simulink model "Citation"  (Simulink 9.1)
settings: Solver=ode5  StartTime=0.0  StopTime=100  FixedStep=0.01  RelTol=1e-3  EnableMultiTasking=on
values from neighbouring files (symbols this model uses):
  T0 = 288.15    [rho_test.m]
  Vw915 = 0    [initcit.m]
  winddir = 45*(pi/180)    (= 0.785398163397)    [initcit.m]
  x0 = []    [cessnac550_3d_sfnc.m]    (also in sfunxyauto.m)
undefined symbols (not defined in the file or in its folder): chord, cv1, cv2, cv3, cv4, deltagmax1, deltagmax2, deltagmax3, deltagmax4, Deng, ealphag, ealphas, g0, hDME, hGS, kt1, kt2, kt3, lh, massinit, matbuaf, matdaf, matdam, matdbbf, matdeaf, matdgaf, matdqaf, matduaf, matdwaw, matedhr, mateif, matelhr, matemhr, matemv1, matemv2, matemve, matetam, mateuaf, matfaaf, matfaxl, matff, matibaf, matibmh, matipaf, matipmh, matiraf, matiuaf, matiwaf, matlaf, matlam, matleaf, matleam, matlgaf, matlqaf, matluaf, matmaaf, matmaam, matmaf, matmam, matmbbf ... (+74)
undefined symbols (not defined in the file): matibb
libraries: vrlib x1
(part 1 of 4)
settings Model: Creator=laurensvaneykeren  LastModifiedBy=jelle  ExtModeTrigMode=oneshot  ExtModeArmWhenConnect=off
settings DataIOCC: SignalLoggingSaveFormat=ModelDataLogs  SignalLoggingName=sigsOut
settings OptimizationCC: BooleanDataType=off  ExpressionDepthLimit=2147483647
settings DebuggingCC: SaveWithParameterizedLinksMsg=none  SignalResolutionControl=TryResolveAllWithWarning  MultiTaskDSMMsg=warning  MultiTaskCondExecSysMsg=none  FcnCallInpInsideContextMsg=warning  StateNameClashWarn=warning
settings HardwareCC: TargetUnknown=on
settings RTWCC: SystemTargetFile=grt_malloc.tlc  GenCodeOnly=on  TemplateMakefile=grt_malloc_default_tmf
settings GRTTargetCC: UseMalloc=on

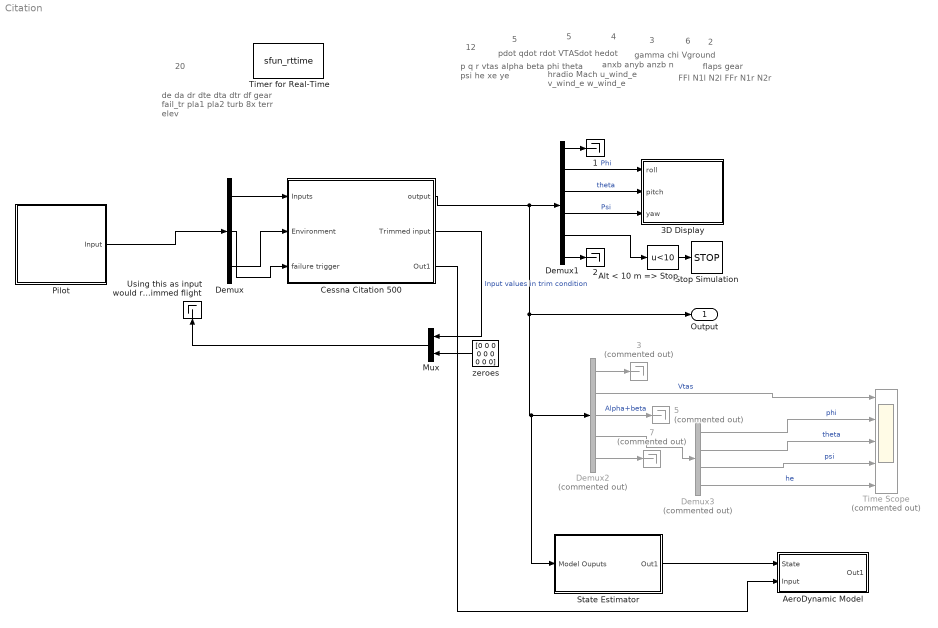
== system Citation ==
  note: de
      | da
      | dr
      | dte
      | dta
      | dtr
      | df
      | gear
      | fail_tr
      | pla1
      | pla2
      | turb 8x
      | terr elev
  note: p
      | q
      | r
      | vtas
      | alpha
      | beta
      | phi
      | theta
      | psi
      | he
      | xe
      | ye
  note: pdot
      | qdot
      | rdot
      | VTASdot
      | hedot
  note: hradio
      | Mach
      | u_wind_e
      | v_wind_e
      | w_wind_e
  note: anxb
      | anyb
      | anzb
      | n
  note: gamma
      | chi
      | Vground
  note: flaps
      | gear
  note: FFl
      | N1l
      | N2l
      | FFr
      | N1r
      | N2r
  note: 12
  note: 5
  note: 5
  note: 4
  note: 3
  note: 6
  note: 2
  note: 20
  1 : Terminator
  2 : Terminator
  3 : Terminator  Commented=on
  3D Display : Subsystem
  5 : Terminator  Commented=on
  7 : Terminator  Commented=on
  "AeroDynamic Model " : Subsystem
  Alt < 10 m => Stop : Fcn  Expr=u<10
  Cessna Citation 500 : Subsystem  mask(Citation Aircraft Model){trimdatafile=example.tri}
      mask prompts: trimdatafile "Trim Condition"
      mask init:
      | initcit;
      mask Display:
      | image(imread('Citation.jpg'))
      | port_label('input', 1, 'Inputs')
      | port_label('input', 2, 'Environment')
      | port_label('output', 1, 'Outputs')
      | port_label('output', 2, 'Trim inputs')
  Demux : Demux  Outputs=[10 1 9]
  Demux1 : Demux  Outputs=[6 1 1 1 1 27]
  Demux2 : Demux  Commented=on  Outputs=[3 1 2 4 27]
  Demux3 : Demux  Commented=on
  Mux : Mux  Inputs=2
  Pilot : Subsystem
  "State Estimator " : Subsystem
  Stop Simulation : Stop
  Time Scope : Scope  Commented=on  NumInputPorts=5
  Timer for Real-Time : S-Function  FunctionName=sfun_rttime  Parameters=1  SFunctionDeploymentMode=off  EnableBusSupport=off
  Using this as input would result in  trimmed flight : Terminator
  zeroes : Constant  Value=[0 0 0 0 0 0 0 0 0]
  Output : Outport
  wires:
  Demux/1 -> Cessna Citation 500/1(Inputs)
  Pilot/1(Input) -> Demux/1
  Cessna Citation 500/1(output) -> Demux1/1, "State Estimator "/1(Model Ouputs), Demux2/1, Output/1
  Demux/3 -> Cessna Citation 500/2(Environment)
  Cessna Citation 500/2(Trimmed input) -> Mux/1  "Input values in trim condition"
  zeroes/1 -> Mux/2
  Mux/1 -> Using this as input would result in  trimmed flight/1
  Demux1/1 -> 1/1
  Demux1/5 -> Alt < 10 m => Stop/1
  Demux1/2 -> 3D Display/1(roll)  "Phi"
  Demux1/3 -> 3D Display/2(pitch)  "theta"
  Demux1/4 -> 3D Display/3(yaw)  "Psi"
  Alt < 10 m => Stop/1 -> Stop Simulation/1
  Demux1/6 -> 2/1
  Demux/2 -> Cessna Citation 500/3("failure trigger ")
  Demux2/1 -> 3/1
  Demux2/2 -> Time Scope/1  "Vtas"
  Demux2/3 -> 5/1  "Alpha+beta"
  Demux2/4 -> Demux3/1
  Demux2/5 -> 7/1
  Demux3/1 -> Time Scope/2  "phi"
  Demux3/2 -> Time Scope/3  "theta"
  Demux3/3 -> Time Scope/4  "psi"
  Demux3/4 -> Time Scope/5  "he"
  "State Estimator "/1(Out1) -> "AeroDynamic Model "/1(State)
  Cessna Citation 500/3(Out1) -> "AeroDynamic Model "/2(Input)

== system Citation/3D Display ==
  roll : Inport
  pitch : Inport  Port=2
  yaw : Inport  Port=3
  Mux1 : Mux
  Position : Subsystem
  S-Function : S-Function  FunctionName=cessnac550_3d_sfnc  SFunctionDeploymentMode=off  EnableBusSupport=off
  Stop Simulation : Stop
  wires:
  roll/1 -> Mux1/1
  Position/1(Out1) -> Mux1/4
  pitch/1 -> Mux1/2
  yaw/1 -> Mux1/3
  Mux1/1 -> S-Function/1
  S-Function/1 -> Stop Simulation/1

== system Citation/AeroDynamic Model  ==
  note: anxb
      | anyb
      | anzb
      | n
  note: hradio
      | Mach
      | u_wind_e
      | v_wind_e
      | w_wind_e
  note: p
      | q
      | r
      | vtas
      | alpha
      | beta
      | phi
      | theta
      | psi
      | he
      | xe
      | ye
  note: gamma
      | chi
      | Vground
  note: pdot
      | qdot
      | rdot
      | VTASdot
      | hedot
  note: FFl
      | N1l
      | N2l
      | FFr
      | N1r
      | N2r
  note: flaps
      | gear
  note: 6
  note: 5
  note: 12
  note: 3
  note: 5
  note: 4
  note: 2
  note: CX
      | CY
      | CZ
  note: 3
  State : Inport
  Input : Inport  Port=2
  Aerodynamic Forces : Subsystem
  Calculate Air Density : MATLAB Function  TreatAsAtomicUnit=on
  Constant : Constant  Value=massinit
  Demux : Demux  Outputs=[9 1 27]
  Demux1 : Demux  Outputs=[12 4 11]
  Demux2 : Demux  Outputs=[1 7]
  Demux3 : Demux  Outputs=[3 1 5]
  Dynamic Pressure : Subsystem
  Terminator{,2..6} (6 alike) : Terminator
  Wing Area : Constant  Value=S
  Out1 : Outport
  wires:
  State/1 -> Demux/1
  Demux/1 -> Demux3/1
  Demux/2 -> Calculate Air Density/1(h)
  Demux/3 -> Demux1/1
  Demux1/1 -> Terminator2/1
  Demux1/3 -> Terminator3/1
  Constant/1 -> Demux2/1
  Demux2/2 -> Terminator4/1
  Demux1/2 -> Aerodynamic Forces/1(Accelerations)
  Demux3/1 -> Terminator5/1
  Demux3/3 -> Terminator6/1
  Aerodynamic Forces/1(Out1) -> Terminator/1
  Calculate Air Density/1(rho) -> Dynamic Pressure/2(air density)
  Demux3/2 -> Dynamic Pressure/1(Vtas)
  Demux2/1 -> Aerodynamic Forces/4(mass)
  Wing Area/1 -> Aerodynamic Forces/3(S)
  Dynamic Pressure/1(Out1) -> Aerodynamic Forces/2(q)

== system Citation/Cessna Citation 500 ==
  note: output is actuator deflection before failure
  note: p
      | q
      | r
      | vtas
      | alpha
      | beta
      | phi
      | theta
      | psi
      | he
      | xe
      | ye
  note: de
      | da
      | dr
      | dte
      | dta
      | dtr
      | df
      | gear
      | pla1
      | pla2
  note: pdot
      | qdot
      | rdot
      | VTASdot
      | hedot
  note: hradio
      | Mach
      | u_wind_e
      | v_wind_e
      | w_wind_e
  note: anxb
      | anyb
      | anzb
      | n
  note: gamma
      | chi
      | Vground
  note: turb 8x
      | terr_elev
  note: flaps
      | gear
  note: de
      | da
      | dr
      | dte
      | dta
      | dtr
      | df
      | gear
      | pla1
      | pla2
  note: FFl
      | N1l
      | N2l
      | FFr
      | N1r
      | N2r
  note: fail_aileron
  Inputs : Inport
  Environment : Inport  Port=2
  "failure trigger " : Inport  Port=3
  Actuators : Subsystem
  Citation model DASMAT : Subsystem
  Controllers : Subsystem
  Demux4 : Demux  Outputs=[8 2]
  Mux1 : Mux  Inputs=7
  Mux2 : Mux  Inputs=2
  trim conditions : Subsystem
  ua sel : Selector  IndexOptions=Index vector (dialog)  Indices=[5 6]  OutputSizes=1
  xdot sel : Selector  IndexOptions=Index vector (dialog)  Indices=[1 2 3 4 10]  OutputSizes=1
  yacc sel : Selector  IndexOptions=Index vector (dialog)  Indices=[4 5 6 15]  OutputSizes=1
  yair sel : Selector  IndexOptions=Index vector (dialog)  Indices=[6 9 22 23 24]  OutputSizes=1
  yfp sel : Selector  IndexOptions=Index vector (dialog)  Indices=[1 2 15]  OutputSizes=1
  ypp sel : Selector  IndexOptions=Index vector (dialog)  Indices=[2 3 4 13 14 15]  OutputSizes=1
  output : Outport
  Trimmed input : Outport  Port=2
  Out1 : Outport  Port=3
  wires:
  Mux1/1 -> output/1
  Citation model DASMAT/1(x) -> Mux1/1, Controllers/1(state)
  Inputs/1 -> Controllers/2(inputs)
  Demux4/1 -> Citation model DASMAT/1(ua), ua sel/1
  Demux4/2 -> Citation model DASMAT/2(ut)
  Environment/1 -> Citation model DASMAT/3(Environment)
  Citation model DASMAT/3(yair) -> yair sel/1
  yair sel/1 -> Mux1/3
  Citation model DASMAT/2(xdot) -> xdot sel/1
  xdot sel/1 -> Mux1/2
  yacc sel/1 -> Mux1/4
  Citation model DASMAT/4(yacc) -> yacc sel/1
  yfp sel/1 -> Mux1/5
  Citation model DASMAT/5(yfp) -> yfp sel/1
  Actuators/1(Actuator_True) -> Demux4/1
  trim conditions/1(ua) -> Mux2/1
  trim conditions/2(ut) -> Mux2/2
  Mux2/1 -> Trimmed input/1
  Controllers/1(control inputs) -> Actuators/1(In)
  ua sel/1 -> Mux1/7
  Citation model DASMAT/6(ypp) -> ypp sel/1
  ypp sel/1 -> Mux1/6
  "failure trigger "/1 -> Actuators/2("failure trigger ")
  Actuators/2(Actuator_est) -> Out1/1

== system Citation/Pilot ==
  note: de
      | da
      | dr
      | dte
      | dta
      | dtr
      | df
      | gear
      | pla1
      | pla2
      | failure_tr
      | turb 8x
      | terr elev
  Joystick : Subsystem
  Mux : Mux  Inputs=13
  "button2toggle " : Subsystem
  da trim : Constant  Value=0
  de trim : Constant  Value=0
  delta flaps : Constant  Value=0
  dr trim : Constant  Value=0
  gear (ON=1/OFF=0) : Constant  Value=0
  terr elev : Constant  Value=0
  turb 8x : Constant  Value=zeros(1,8)
  Input : Outport
  wires:
  Mux/1 -> Input/1
  Joystick/1(delta elevator) -> Mux/1
  Joystick/3(delta rudder) -> Mux/3
  da trim/1 -> Mux/5
  de trim/1 -> Mux/4
  Joystick/2(delta aileron) -> Mux/2
  turb 8x/1 -> Mux/12
  terr elev/1 -> Mux/13
  Joystick/4(Throttle setting) -> Mux/10, Mux/9
  gear (ON=1/OFF=0)/1 -> Mux/8
  dr trim/1 -> Mux/6
  delta flaps/1 -> Mux/7
  Joystick/5("Failure buttons ") -> "button2toggle "/1(In1)
  "button2toggle "/1(Out1) -> Mux/11

== system Citation/State Estimator  ==
  note: It is assumed that the model ouputs are perfect measurements
  Model Ouputs : Inport
  Out1 : Outport
  wires:
  Model Ouputs/1 -> Out1/1

== system Citation/3D Display/Position ==
  Mux2 : Mux  Inputs=3
  x : Constant  Value=0
  y : Constant  Value=0
  z : Constant  Value=0
  Out1 : Outport
  wires:
  y/1 -> Mux2/2
  z/1 -> Mux2/3
  x/1 -> Mux2/1
  Mux2/1 -> Out1/1

== system Citation/AeroDynamic Model /Aerodynamic Forces ==
  note: accelerations are given in [g]
  note: anxb
      | anyb
      | anzb
      | n
  Accelerations : Inport
  q : Inport  Port=2
  S : Inport  Port=3
  mass : Inport  Port=4
  Demux : Demux  Outputs=[3 1]
  Divide : Product  Inputs=*/
  Gain : Gain  Gain=g0
  Product : Product
  Product2 : Product
  Terminator : Terminator
  Out1 : Outport
  wires:
  Accelerations/1 -> Demux/1
  Demux/2 -> Terminator/1
  Demux/1 -> Gain/1
  Gain/1 -> Product2/1
  mass/1 -> Product2/2
  q/1 -> Product/1
  S/1 -> Product/2
  Product2/1 -> Divide/1
  Divide/1 -> Out1/1
  Product/1 -> Divide/2

== system Citation/AeroDynamic Model /Dynamic Pressure ==
  Vtas : Inport
  air density : Inport  Port=2
  Gain : Gain  Gain=0.5
  Product : Product
  Product1 : Product
  Out1 : Outport
  wires:
  Vtas/1 -> Product/2, Product/1
  air density/1 -> Product1/2
  Product/1 -> Product1/1
  Gain/1 -> Out1/1
  Product1/1 -> Gain/1

== system Citation/Cessna Citation 500/Actuators ==
  note: de
      | da
      | dr
      | dte
      | dta
      | dtr
      | df
      | gear
      | pla1
      | pla2
  note: de
      | da
      | dr
      | dte
      | dta
      | dtr
      | df
      | gear
      | pla1
      | pla2
  In : Inport
  "failure trigger " : Inport  Port=2
  Demux : Demux  Outputs=10
  Demux1 : Demux  Outputs=[1 1 8]
  Gain : Gain  Gain=0.5
  Mux : Mux  Inputs=10
  Mux1 : Mux  Inputs=3
  Sum : Sum  Inputs=|++
  Switch : Switch  Criteria=u2 > Threshold
  Terminator : Terminator
  "aileron failure offset (deg) " : Constant  Value=16
  da : Subsystem
  da limits : Saturate  UpperLimit=0.65  LowerLimit=-0.65
  de : Subsystem
  de limits : Saturate  UpperLimit=0.26  LowerLimit=-0.35
  deg2rad : Gain  Gain=pi/180
  dr : Subsystem
  dr limits : Saturate  UpperLimit=0.38  LowerLimit=-0.38
  flaps : Subsystem
  gear : Subsystem
  Actuator_True : Outport
  Actuator_est : Outport  Port=2
  wires:
  In/1 -> Demux/1
  Mux/1 -> Demux1/1, Actuator_True/1
  Demux/1 -> de/1(In)
  Demux/2 -> da/1(In)
  Demux/3 -> dr/1(In)
  de/1(Out) -> de limits/1
  da/1(Out) -> da limits/1
  dr/1(Out) -> dr limits/1
  dr limits/1 -> Mux/3
  de limits/1 -> Mux/1
  Demux/8 -> gear/1(In)
  Demux/7 -> flaps/1(In)
  Demux/9 -> Mux/9
  Demux/10 -> Mux/10
  flaps/1(Out) -> Mux/7
  gear/1(Out) -> Mux/8
  Demux/4 -> Mux/4
  Demux/5 -> Mux/5
  Demux/6 -> Mux/6
  da limits/1 -> Gain/1, Switch/3, Mux1/2
  "failure trigger "/1 -> Switch/2
  "aileron failure offset (deg) "/1 -> deg2rad/1
  deg2rad/1 -> Sum/1
  Gain/1 -> Sum/2
  Sum/1 -> Switch/1
  Switch/1 -> Mux/2
  Demux1/2 -> Terminator/1
  Demux1/1 -> Mux1/1
  Demux1/3 -> Mux1/3
  Mux1/1 -> Actuator_est/1

== system Citation/Cessna Citation 500/Citation model DASMAT ==
  ua : Inport
  ut : Inport  Port=2
  Environment : Inport  Port=3
  AIRCRAFT MODEL : Subsystem
  Mux1 : Mux  Inputs=[8 2 8 12 8]
  Terminator_{16..19} (4 alike) : Terminator
  massinit : Constant  Value=massinit
  x : Outport
  xdot : Outport  Port=2
  yair : Outport  Port=3
  yacc : Outport  Port=4
  yfp : Outport  Port=5
  ypp : Outport  Port=6
  wires:
  AIRCRAFT MODEL/13(FMt) -> Terminator_19/1
  Mux1/1 -> yair/1
  AIRCRAFT MODEL/12(FMag) -> Terminator_17/1
  AIRCRAFT MODEL/11(FMa) -> Terminator_18/1
  AIRCRAFT MODEL/7(gust) -> Mux1/5
  AIRCRAFT MODEL/6(wind) -> Mux1/4
  AIRCRAFT MODEL/5(yad2) -> Mux1/3
  AIRCRAFT MODEL/4(yad1) -> Mux1/2
  AIRCRAFT MODEL/3(yatm) -> Mux1/1
  AIRCRAFT MODEL/2(xdot) -> xdot/1
  AIRCRAFT MODEL/1(x) -> x/1
  AIRCRAFT MODEL/10(ys) -> Terminator_16/1
  AIRCRAFT MODEL/9(yfp) -> yfp/1
  AIRCRAFT MODEL/8(yacc) -> yacc/1
  massinit/1 -> AIRCRAFT MODEL/3(massinit)
  ut/1 -> AIRCRAFT MODEL/2(ut)
  ua/1 -> AIRCRAFT MODEL/1(ua)
  Environment/1 -> AIRCRAFT MODEL/4(Environment)
  AIRCRAFT MODEL/14(ypp) -> ypp/1

== system Citation/Cessna Citation 500/Controllers ==
  state : Inport
  inputs : Inport  Port=2
  A/T disabled : Gain  Gain=0  SaturateOnIntegerOverflow=on  OutDataTypeStr=Inherit: Same as input  ParamDataTypeStr=Inherit: Same as input
  Yaw damper : Subsystem
  add controller outputs to pilot inputs : Sum  Inputs=|+|+|+|  SaturateOnIntegerOverflow=on
  auto throttle : Subsystem
  control inputs : Outport
  wires:
  state/1 -> Yaw damper/1(state), auto throttle/1(state)
  inputs/1 -> Yaw damper/2(inputs), add controller outputs to pilot inputs/3, auto throttle/2(inputs)
  add controller outputs to pilot inputs/1 -> control inputs/1
  Yaw damper/1(controller output) -> add controller outputs to pilot inputs/1
  auto throttle/1(controller output) -> A/T disabled/1
  A/T disabled/1 -> add controller outputs to pilot inputs/2

== system Citation/Cessna Citation 500/trim conditions ==
  PLA1/Tx1 : Constant  Value=ut0(1)
  PLA2/Tx2 : Constant  Value=ut0(2)
  control inputs : Mux  Inputs=8
      settings: DisplayOption=signals
  deltaa : Constant  Value=u0(2)
  deltae : Constant  Value=u0(1)
  deltaf : Constant  Value=u0(7)
  deltar : Constant  Value=u0(3)
  deltata : Constant  Value=u0(5)
  deltate : Constant  Value=u0(4)
  deltatr : Constant  Value=u0(6)
  engine inputs : Mux  Inputs=2
      settings: DisplayOption=signals
  lgsw : Constant  Value=u0(8)
  ua : Outport
  ut : Outport  Port=2
  wires:
  deltaf/1 -> control inputs/7  "df"
  engine inputs/1 -> ut/1
  deltatr/1 -> control inputs/6  "dtr"
  deltata/1 -> control inputs/5  "dta"
  control inputs/1 -> ua/1
  PLA1/Tx1/1 -> engine inputs/1  "pla1"
  PLA2/Tx2/1 -> engine inputs/2  "pla2"
  deltae/1 -> control inputs/1  "de"
  deltaa/1 -> control inputs/2  "da"
  deltar/1 -> control inputs/3  "dr"
  deltate/1 -> control inputs/4  "dte"
  lgsw/1 -> control inputs/8  "lg"

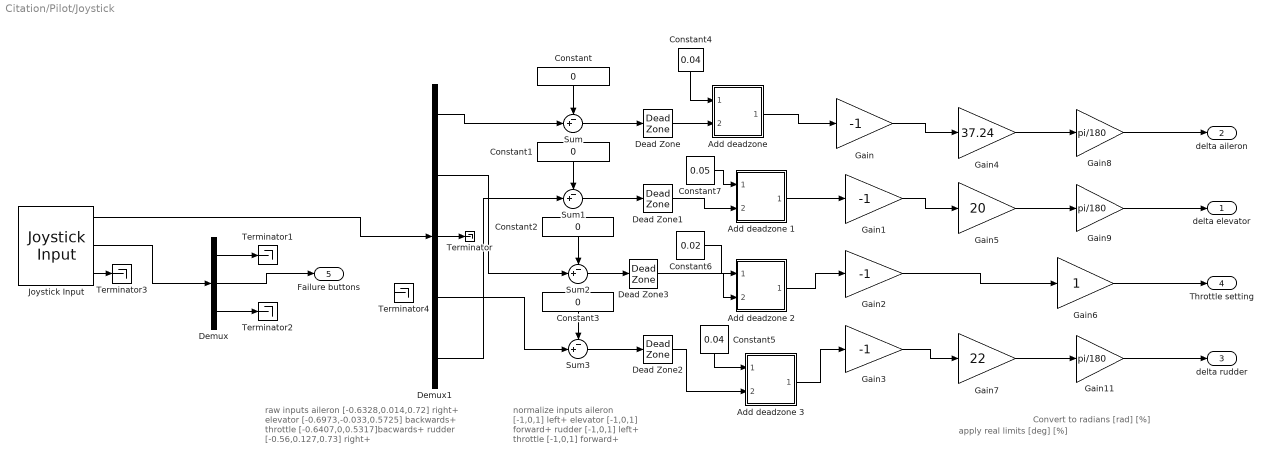
== system Citation/Pilot/Joystick ==
  note: raw inputs
      | aileron [-0.6328,0.014,0.72] right+
      | elevator [-0.6973,-0.033,0.5725] backwards+
      | throttle [-0.6407,0,0.5317]bacwards+
      | rudder [-0.56,0.127,0.73] right+
  note: normalize inputs
      | aileron [-1,0,1] left+
      | elevator [-1,0,1] forward+
      | rudder [-1,0,1] left+
      | throttle [-1,0,1] forward+
  note: apply real limits
      | [deg]
      | [%]
  note: Convert to radians
      | [rad]
      | [%]
  "Add deadzone " : Subsystem
  Add deadzone 1 : Subsystem
  Add deadzone 2 : Subsystem
  Add deadzone 3 : Subsystem
  Constant{,1..3} (4 alike) : Constant  Value=0
  Constant4 : Constant  Value=0.04
  Constant5 : Constant  Value=0.04
  Constant6 : Constant  Value=0.02
  Constant7 : Constant  Value=0.05
  Dead Zone : DeadZone  LowerValue=-0.04  UpperValue=0.04  SaturateOnIntegerOverflow=on
  Dead Zone1 : DeadZone  LowerValue=-0.05  UpperValue=0.05  SaturateOnIntegerOverflow=on
  Dead Zone2 : DeadZone  LowerValue=-0.04  UpperValue=0.04  SaturateOnIntegerOverflow=on
  Dead Zone3 : DeadZone  LowerValue=-0.02  UpperValue=0.02  SaturateOnIntegerOverflow=on
  Demux : Demux  Outputs=[2 1 7]
  Demux1 : Demux  Outputs=5
  Gain{,1..3} (4 alike) : Gain  Gain=-1  SaturateOnIntegerOverflow=on  OutDataTypeStr=Inherit: Same as input  ParamDataTypeStr=Inherit: Same as input
  Gain11 : Gain  Gain=pi/180  SaturateOnIntegerOverflow=on  OutDataTypeStr=Inherit: Same as input  ParamDataTypeStr=Inherit: Same as input
  Gain4 : Gain  Gain=37.24  SaturateOnIntegerOverflow=on  OutDataTypeStr=Inherit: Same as input  ParamDataTypeStr=Inherit: Same as input
  Gain5 : Gain  Gain=20  SaturateOnIntegerOverflow=on  OutDataTypeStr=Inherit: Same as input  ParamDataTypeStr=Inherit: Same as input
  Gain6 : Gain  SaturateOnIntegerOverflow=on  OutDataTypeStr=Inherit: Same as input  ParamDataTypeStr=Inherit: Same as input
  Gain7 : Gain  Gain=22  SaturateOnIntegerOverflow=on  OutDataTypeStr=Inherit: Same as input  ParamDataTypeStr=Inherit: Same as input
  Gain8 : Gain  Gain=pi/180  SaturateOnIntegerOverflow=on  OutDataTypeStr=Inherit: Same as input  ParamDataTypeStr=Inherit: Same as input
  Gain9 : Gain  Gain=pi/180  SaturateOnIntegerOverflow=on  OutDataTypeStr=Inherit: Same as input  ParamDataTypeStr=Inherit: Same as input
  Joystick Input : vrlib/Joystick Input  joyid=1  adjustports=on  forcefeed=off
      settings: SourceProductBaseCode=VR
  Sum{,1..3} (4 alike) : Sum  Inputs=-+|  SaturateOnIntegerOverflow=on
  Terminator{,1..4} (5 alike) : Terminator
  delta elevator : Outport
  delta aileron : Outport  Port=2
  delta rudder : Outport  Port=3
  Throttle setting : Outport  Port=4
  "Failure buttons " : Outport  Port=5
  wires:
  Joystick Input/1 -> Demux1/1
  Joystick Input/2 -> Demux/1
  ? -> Terminator4/1
  Demux1/1 -> Sum/2
  Constant/1 -> Sum/1
  Constant1/1 -> Sum1/1
  Constant2/1 -> Sum2/1
  Constant3/1 -> Sum3/1
  Sum/1 -> Dead Zone/1
  Gain/1 -> Gain4/1
  Sum1/1 -> Dead Zone1/1
  Gain1/1 -> Gain5/1
  Sum3/1 -> Dead Zone2/1
  Gain3/1 -> Gain7/1
  Gain4/1 -> Gain8/1
  Gain5/1 -> Gain9/1
  Gain6/1 -> Throttle setting/1
  Gain7/1 -> Gain11/1
  Gain8/1 -> delta aileron/1
  Gain9/1 -> delta elevator/1
  Gain11/1 -> delta rudder/1
  Gain2/1 -> Gain6/1
  Demux1/5 -> Sum1/2
  Demux1/4 -> Sum3/2
  Demux1/2 -> Sum2/2
  Demux1/3 -> Terminator/1
  Constant4/1 -> "Add deadzone "/1("Value  ")
  Dead Zone/1 -> "Add deadzone "/2("Input ")
  Dead Zone1/1 -> Add deadzone 1/2("Input ")
  Constant5/1 -> Add deadzone 3/1("Value  ")
  Dead Zone2/1 -> Add deadzone 3/2("Input ")
  Add deadzone 3/1(Out1) -> Gain3/1
  Add deadzone 2/1(Out1) -> Gain2/1
  Add deadzone 1/1(Out1) -> Gain1/1
  "Add deadzone "/1(Out1) -> Gain/1
  Sum2/1 -> Dead Zone3/1
  Dead Zone3/1 -> Add deadzone 2/2("Input ")
  Constant6/1 -> Add deadzone 2/1("Value  ")
  Constant7/1 -> Add deadzone 1/1("Value  ")
  Demux/1 -> Terminator1/1
  Demux/3 -> Terminator2/1
  Demux/2 -> "Failure buttons "/1
  Joystick Input/3 -> Terminator3/1

== system Citation/Pilot/button2toggle  ==
  In1 : Inport
  Constant1 : Constant
  Constant2 : Constant  Value=0
  Memory : Memory
  Switch : Switch  Criteria=u2 > Threshold
  Triggered Subsystem : Subsystem  TreatAsAtomicUnit=on
  Out1 : Outport
  wires:
  Memory/1 -> Switch/2
  Switch/1 -> Triggered Subsystem/1(In1)
  Constant2/1 -> Switch/1
  In1/1 -> Triggered Subsystem/Trigger
  Constant1/1 -> Switch/3
  Triggered Subsystem/1(Out1) -> Out1/1, Memory/1

== system Citation/Cessna Citation 500/Actuators/da ==
  In : Inport
  Gain : Gain  Gain=13  SaturateOnIntegerOverflow=on  OutDataTypeStr=Inherit: Same as input  ParamDataTypeStr=Inherit: Same as input
  Integrator : Integrator  InitialCondition=u0(2)
  Sum : Sum  Inputs=|+-  SaturateOnIntegerOverflow=on
  Out : Outport
  wires:
  Integrator/1 -> Out/1, Sum/2
  In/1 -> Sum/1
  Sum/1 -> Gain/1
  Gain/1 -> Integrator/1

== system Citation/Cessna Citation 500/Actuators/de ==
  In : Inport
  Gain : Gain  Gain=13  SaturateOnIntegerOverflow=on  OutDataTypeStr=Inherit: Same as input  ParamDataTypeStr=Inherit: Same as input
  Integrator : Integrator  InitialCondition=u0(1)
  Sum : Sum  Inputs=|+-  SaturateOnIntegerOverflow=on
  Out : Outport
  wires:
  Integrator/1 -> Out/1, Sum/2
  In/1 -> Sum/1
  Sum/1 -> Gain/1
  Gain/1 -> Integrator/1

== system Citation/Cessna Citation 500/Actuators/dr ==
  In : Inport
  Gain : Gain  Gain=13  SaturateOnIntegerOverflow=on  OutDataTypeStr=Inherit: Same as input  ParamDataTypeStr=Inherit: Same as input
  Integrator : Integrator  InitialCondition=u0(3)
  Sum : Sum  Inputs=|+-  SaturateOnIntegerOverflow=on
  Out : Outport
  wires:
  Integrator/1 -> Out/1, Sum/2
  In/1 -> Sum/1
  Sum/1 -> Gain/1
  Gain/1 -> Integrator/1

== system Citation/Cessna Citation 500/Actuators/flaps ==
  In : Inport
  Gain : Gain  Gain=0.9  SaturateOnIntegerOverflow=on  OutDataTypeStr=Inherit: Same as input  ParamDataTypeStr=Inherit: Same as input
  Integrator : Integrator  InitialCondition=u0(7)
  Sum : Sum  Inputs=|+-  SaturateOnIntegerOverflow=on
  Out : Outport
  wires:
  Integrator/1 -> Out/1, Sum/2
  In/1 -> Sum/1
  Sum/1 -> Gain/1
  Gain/1 -> Integrator/1

== system Citation/Cessna Citation 500/Actuators/gear ==
  In : Inport
  Gain : Gain  Gain=0.6  SaturateOnIntegerOverflow=on  OutDataTypeStr=Inherit: Same as input  ParamDataTypeStr=Inherit: Same as input
  Integrator : Integrator  InitialCondition=u0(8)
  Sum : Sum  Inputs=|+-  SaturateOnIntegerOverflow=on
  Out : Outport
  wires:
  Integrator/1 -> Out/1, Sum/2
  In/1 -> Sum/1
  Sum/1 -> Gain/1
  Gain/1 -> Integrator/1

== system Citation/Cessna Citation 500/Citation model DASMAT/AIRCRAFT MODEL ==
  ua : Inport
  ut : Inport  Port=2
  massinit : Inport  Port=3
  Environment : Inport  Port=4
  AFM : Subsystem
  AIRDATA : Subsystem
  Demux : Demux  Outputs=[8 1]
  EFM : Subsystem
  EQM : Subsystem
  FM SORT : Subsystem
  GRAVITY : Subsystem
  LANDING GEAR : Subsystem
  OBSERVATIONS : Subsystem
  WIND/TURBULENCE : Subsystem
  x : Outport
  xdot : Outport  Port=2
  yatm : Outport  Port=3
  yad1 : Outport  Port=4
  yad2 : Outport  Port=5
  wind : Outport  Port=6
  gust : Outport  Port=7
  yacc : Outport  Port=8
  yfp : Outport  Port=9
  ys : Outport  Port=10
  FMa : Outport  Port=11
  FMag : Outport  Port=12
  FMt : Outport  Port=13
  ypp : Outport  Port=14
  wires:
  AFM/1(FMa) -> FM SORT/1(FMa), EQM/2(FMa)
  OBSERVATIONS/3(ys) -> ys/1
  OBSERVATIONS/2(yfp) -> yfp/1
  EQM/4(FMtot corrected) -> OBSERVATIONS/4(FMtot)
  EQM/3(yuvw) -> OBSERVATIONS/3(yuvw)
  EFM/1(FMt) -> FM SORT/3(FMt), FMt/1
  AFM/4(FMag) -> FM SORT/2(FMag), FMag/1
  ua/1 -> AFM/2(ua), LANDING GEAR/4(ua)
  ut/1 -> EFM/2(ut)
  OBSERVATIONS/1(yacc) -> yacc/1
  FM SORT/1(FMtot) -> EQM/1("FMtot ")
  EQM/5(FMa corrected) -> OBSERVATIONS/5(FMa), FMa/1
  AFM/2(FMadot) -> EQM/3(FMadot)
  AFM/3(FMbdot) -> EQM/4(FMbdot)
  GRAVITY/1(Fgr) -> FM SORT/4("Fgr "), OBSERVATIONS/6(Fgr)
  massinit/1 -> EFM/3(massinit), AFM/3(massinit), GRAVITY/2(massinit), EQM/5(massinit), OBSERVATIONS/7(massinit), LANDING GEAR/3(massinit)
  AIRDATA/3(yad2) -> EFM/6(yad2), AFM/5(yad2), yad2/1
  AIRDATA/2(yad1) -> AFM/4(yad1), EFM/5(yad1), yad1/1
  AIRDATA/1(yatm) -> yatm/1, GRAVITY/3(yatm), OBSERVATIONS/8(yatm), EFM/4(yatm), AFM/7(yatm)
  EQM/1(x) -> GRAVITY/1("x "), LANDING GEAR/1(x), EFM/1(x), AFM/1(x), WIND/TURBULENCE/1("x "), AIRDATA/1(x), x/1, OBSERVATIONS/1(x)
  WIND/TURBULENCE/1(wind) -> EQM/6(wind), wind/1
  EQM/2(xdot) -> xdot/1, OBSERVATIONS/2(xdot), LANDING GEAR/2(xdot)
  Environment/1 -> Demux/1
  Demux/1 -> gust/1, AFM/6(gust)
  Demux/2 -> AIRDATA/2(terrain  elevation), LANDING GEAR/5(terr elev)  "terrain elevation"
  LANDING GEAR/1(Fmt) -> FM SORT/5(Fgear)
  EFM/2(ypp) -> ypp/1

== system Citation/Cessna Citation 500/Controllers/Yaw damper ==
  state : Inport
  inputs : Inport  Port=2
  Gain : Gain  SaturateOnIntegerOverflow=on  OutDataTypeStr=Inherit: Same as input  ParamDataTypeStr=Inherit: Same as input
  Washout : TransferFcn  Numerator=[1 0]  Denominator=[1 1/4]
  dr : Gain  Gain=[0 0 1 0 0 0 0 0 0 0]  SaturateOnIntegerOverflow=on  OutDataTypeStr=Inherit: Same as input  ParamDataTypeStr=Inherit: Same as input
  not used : Terminator
  r  sel : Selector  IndexOptions=Index vector (dialog)  Indices=[3]  OutputSizes=1
  controller output : Outport
  wires:
  Washout/1 -> Gain/1
  dr/1 -> controller output/1
  state/1 -> r  sel/1
  r  sel/1 -> Washout/1  "r"
  inputs/1 -> not used/1
  Gain/1 -> dr/1

== system Citation/Cessna Citation 500/Controllers/auto throttle ==
  state : Inport
  inputs : Inport  Port=2
  Gain : Gain  Gain=0.5  SaturateOnIntegerOverflow=on  OutDataTypeStr=Inherit: Same as input  ParamDataTypeStr=Inherit: Same as input
  Saturation : Saturate  UpperLimit=1.0  LowerLimit=0.0
  Sum : Sum  Inputs=+-|  SaturateOnIntegerOverflow=on
  VTAS ref (trim value) : Constant  Value=x0(4)
  VTAS sel : Selector  IndexOptions=Index vector (dialog)  Indices=[4]  OutputSizes=1
  controller output is later added to pilot input! : Sum  Inputs=|+-  SaturateOnIntegerOverflow=on
  pla1&2 : Gain  Gain=[0 0 0 0 0 0 0 0 1 1]  SaturateOnIntegerOverflow=on  OutDataTypeStr=Inherit: Same as input  ParamDataTypeStr=Inherit: Same as input
  pla1&2 as well : Gain  Gain=[0 0 0 0 0 0 0 0 1 1]  SaturateOnIntegerOverflow=on  OutDataTypeStr=Inherit: Same as input  ParamDataTypeStr=Inherit: Same as input
  controller output : Outport
  wires:
  inputs/1 -> pla1&2 as well/1
  state/1 -> VTAS sel/1
  VTAS sel/1 -> Sum/2  "VTAS"
  VTAS ref (trim value)/1 -> Sum/1
  Sum/1 -> Gain/1
  pla1&2/1 -> controller output is later added to pilot input!/1
  Gain/1 -> Saturation/1
  controller output is later added to pilot input!/1 -> controller output/1
  Saturation/1 -> pla1&2/1
  pla1&2 as well/1 -> controller output is later added to pilot input!/2

== system Citation/Pilot/Joystick/Add deadzone  ==
  note: Add or subtract deadzone value
  note: Check sign
  "Value  " : Inport
  "Input " : Inport  Port=2
  Product : Product
  Sign : Signum
  Sum4 : Sum  Inputs=|++
  Out1 : Outport
  wires:
  "Input "/1 -> Sign/1, Sum4/2
  Product/1 -> Sum4/1
  "Value  "/1 -> Product/1
  Sum4/1 -> Out1/1
  Sign/1 -> Product/2

== system Citation/Pilot/Joystick/Add deadzone 1 ==
  note: Check sign
  note: Add or subtract deadzone value
  "Value  " : Inport
  "Input " : Inport  Port=2
  Product : Product
  Sign : Signum
  Sum4 : Sum  Inputs=|++
  Out1 : Outport
  wires:
  Sign/1 -> Product/2
  Sum4/1 -> Out1/1
  "Value  "/1 -> Product/1
  Product/1 -> Sum4/1
  "Input "/1 -> Sum4/2, Sign/1

== system Citation/Pilot/Joystick/Add deadzone 2 ==
  note: Add or subtract deadzone value
  note: Check sign
  "Value  " : Inport
  "Input " : Inport  Port=2
  Product : Product
  Sign : Signum
  Sum4 : Sum  Inputs=|++
  Out1 : Outport
  wires:
  "Input "/1 -> Sign/1, Sum4/2
  Product/1 -> Sum4/1
  "Value  "/1 -> Product/1
  Sum4/1 -> Out1/1
  Sign/1 -> Product/2

== system Citation/Pilot/Joystick/Add deadzone 3 ==
  note: Check sign
  note: Add or subtract deadzone value
  "Value  " : Inport
  "Input " : Inport  Port=2
  Product : Product
  Sign : Signum
  Sum4 : Sum  Inputs=|++
  Out1 : Outport
  wires:
  Sign/1 -> Product/2
  Sum4/1 -> Out1/1
  "Value  "/1 -> Product/1
  Product/1 -> Sum4/1
  "Input "/1 -> Sum4/2, Sign/1

== system Citation/Pilot/button2toggle /Triggered Subsystem ==
  In1 : Inport
  Trigger : TriggerPort  VariantControl=Variant
  Out1 : Outport
  wires:
  In1/1 -> Out1/1

== system Citation/Cessna Citation 500/Citation model DASMAT/AIRCRAFT MODEL/AFM ==
  x : Inport
  ua : Inport  Port=2
  massinit : Inport  Port=3
  yad1 : Inport  Port=4
  yad2 : Inport  Port=5
  gust : Inport  Port=6
  yatm : Inport  Port=7
  Aero axes-cg transformation : Subsystem
  Aeromod : Subsystem
  FMaerodims : Subsystem
  FMgustdims : Subsystem
  Gust axes-cg transformation : Subsystem
  FMa : Outport
  FMadot : Outport  Port=2
  FMbdot : Outport  Port=3
  FMag : Outport  Port=4
  wires:
  FMaerodims/3(FMbdot) -> FMbdot/1
  FMgustdims/1(FMag) -> FMag/1
  FMaerodims/2(FMadot) -> FMadot/1
  FMaerodims/1(FMa) -> FMa/1
  ua/1 -> Aeromod/2(ua)
  yad2/1 -> Aeromod/5(yad2)
  gust/1 -> Aeromod/6(gust)
  Aero axes-cg transformation/1(Ca) -> FMaerodims/1(Ca)
  Aero axes-cg transformation/2(Cadot) -> FMaerodims/2(Cadot)
  Aero axes-cg transformation/3(Cbdot) -> FMaerodims/3(Cbdot)
  Gust axes-cg transformation/1(Cag) -> FMgustdims/1(Cag)
  yad1/1 -> FMaerodims/5(yad1), FMgustdims/2(yad1), Aeromod/4(yad1)
  massinit/1 -> Aero axes-cg transformation/5(massinit), Gust axes-cg transformation/3(massinit), Aeromod/3(massinit)
  Aeromod/1(Ca) -> Aero axes-cg transformation/1(Ca model)
  Aeromod/2(Cadot) -> Aero axes-cg transformation/2(Cadot model)
  Aeromod/3(Cbdot) -> Aero axes-cg transformation/3(Cbdot model)
  Aeromod/4(Cag) -> Gust axes-cg transformation/1(Cag model)
  x/1 -> Aero axes-cg transformation/4("x "), Gust axes-cg transformation/2("x "), FMaerodims/4(x), Aeromod/1(x)
  yatm/1 -> Aeromod/7(yatm)

== system Citation/Cessna Citation 500/Citation model DASMAT/AIRCRAFT MODEL/AIRDATA ==
  x : Inport
  terrain  elevation : Inport  Port=2
  Demux : Demux  Outputs=[8 2 8]
  Demux1 : Demux  Outputs=[5 1 2]
  Demux2 : Demux  Outputs=[1 1 6]
  Mux : Mux  Inputs=[5 1 2]
  Sum : Sum  Inputs=-+|  SaturateOnIntegerOverflow=on
  Terminator : Terminator
  Terminator1 : Terminator
  Time Scope : Scope
  airdata : S-Function  FunctionName=ac_atmos  SFunctionDeploymentMode=off  EnableBusSupport=off
  yatm : Outport
  yad1 : Outport  Port=2
  yad2 : Outport  Port=3
  wires:
  x/1 -> airdata/1
  airdata/1 -> Demux/1
  Demux/2 -> yad1/1
  Demux/3 -> yad2/1
  Demux/1 -> Demux2/1, Demux1/1
  Mux/1 -> yatm/1
  Demux1/1 -> Mux/1
  Demux1/3 -> Mux/3
  Demux1/2 -> Sum/2
  Sum/1 -> Mux/2
  terrain  elevation/1 -> Sum/1
  Demux2/1 -> Terminator/1
  Demux2/2 -> Time Scope/1
  Demux2/3 -> Terminator1/1

== system Citation/Cessna Citation 500/Citation model DASMAT/AIRCRAFT MODEL/EFM ==
  x : Inport
  ut : Inport  Port=2
  massinit : Inport  Port=3
  yatm : Inport  Port=4
  yad1 : Inport  Port=5
  yad2 : Inport  Port=6
  Engine axes-cg transformation : Subsystem
  Engmod : Subsystem
  FMt : Outport
  ypp : Outport  Port=2
  wires:
  massinit/1 -> Engine axes-cg transformation/3(massinit)
  Engine axes-cg transformation/1(FMt) -> FMt/1
  ut/1 -> Engmod/2(ut)
  yatm/1 -> Engmod/3(yatm)
  yad2/1 -> Engmod/5(yad2)
  x/1 -> Engine axes-cg transformation/2("x "), Engmod/1(x)
  yad1/1 -> Engmod/4(yad1)
  Engmod/1(FMt) -> Engine axes-cg transformation/1(FMt model)
  Engmod/2(ypp) -> ypp/1

== system Citation/Cessna Citation 500/Citation model DASMAT/AIRCRAFT MODEL/EQM ==
  "FMtot " : Inport
  FMa : Inport  Port=2
  FMadot : Inport  Port=3
  FMbdot : Inport  Port=4
  massinit : Inport  Port=5
  wind : Inport  Port=6
  CFMa correction : Subsystem
  Integrator : Integrator  InitialCondition=x0
  State Derivatives : Subsystem
  x : Outport
  xdot : Outport  Port=2
  yuvw : Outport  Port=3
  FMtot corrected : Outport  Port=4
  FMa corrected : Outport  Port=5
  wires:
  State Derivatives/2(yuvw) -> yuvw/1
  State Derivatives/3(FMtot corrected) -> FMtot corrected/1
  FMa/1 -> CFMa correction/2(FMa)
  State Derivatives/1(xdot) -> xdot/1, CFMa correction/1(xdot), Integrator/1
  CFMa correction/1(FMa corrected) -> FMa corrected/1
  massinit/1 -> State Derivatives/5(massinit)
  "FMtot "/1 -> State Derivatives/2(FMtot)
  FMadot/1 -> CFMa correction/3(FMadot), State Derivatives/3(FMadot)
  FMbdot/1 -> CFMa correction/4(FMbdot), State Derivatives/4(FMbdot)
  Integrator/1 -> State Derivatives/1(x), x/1
  wind/1 -> State Derivatives/6(wind)

== system Citation/Cessna Citation 500/Citation model DASMAT/AIRCRAFT MODEL/FM SORT ==
  FMa : Inport
  FMag : Inport  Port=2
  FMt : Inport  Port=3
  "Fgr " : Inport  Port=4
  Fgear : Inport  Port=5
  Mux : Mux  Inputs=[12 12]
  Sum : Sum  Inputs=+++++  SaturateOnIntegerOverflow=on  InputSameDT=on  OutDataTypeStr=Inherit: Same as first input
  Sum1 : Sum  Inputs=++++  SaturateOnIntegerOverflow=on  InputSameDT=on  OutDataTypeStr=Inherit: Same as first input
  aero : Demux  Outputs=[12 12]
  engine : Demux  Outputs=[12 12]
  gear : Demux  Outputs=[12 12]
  gust : Demux  Outputs=[12 12]
  FMtot : Outport
  wires:
  FMt/1 -> engine/1
  FMa/1 -> aero/1
  FMag/1 -> gust/1
  gust/2 -> Sum1/2
  Sum1/1 -> Mux/2
  engine/2 -> Sum1/3
  aero/2 -> Sum1/1
  gust/1 -> Sum/2
  engine/1 -> Sum/3
  Sum/1 -> Mux/1
  "Fgr "/1 -> Sum/4
  aero/1 -> Sum/1
  Mux/1 -> FMtot/1
  Fgear/1 -> gear/1
  gear/1 -> Sum/5
  gear/2 -> Sum1/4

== system Citation/Cessna Citation 500/Citation model DASMAT/AIRCRAFT MODEL/GRAVITY ==
  "x " : Inport
  massinit : Inport  Port=2
  yatm : Inport  Port=3
  Fgr transformation : S-Function  FunctionName=ac_axes  Parameters=3  SFunctionDeploymentMode=off  EnableBusSupport=off
  Mux : Mux  Inputs=[12 3]
  Mux1 : Mux  Inputs=3
  Terminator_{1..9} (9 alike) : Terminator
  W : Product  SaturateOnIntegerOverflow=on  InputSameDT=on  OutDataTypeStr=Inherit: Same as first input
  atmosphere : Demux  Outputs=8
  mass cg inertia : Demux  Outputs=[1 3 4]
  zero : Constant  Value=0
  Fgr : Outport
  wires:
  mass cg inertia/3 -> Terminator_9/1
  mass cg inertia/2 -> Terminator_8/1
  atmosphere/8 -> Terminator_7/1
  atmosphere/7 -> Terminator_6/1
  atmosphere/6 -> Terminator_5/1
  atmosphere/5 -> Terminator_4/1
  atmosphere/3 -> Terminator_3/1
  atmosphere/2 -> Terminator_2/1
  atmosphere/1 -> Terminator_1/1
  Mux/1 -> Fgr transformation/1
  "x "/1 -> Mux/1
  Fgr transformation/1 -> Fgr/1
  mass cg inertia/1 -> W/1
  massinit/1 -> mass cg inertia/1
  yatm/1 -> atmosphere/1
  W/1 -> Mux1/3
  Mux1/1 -> Mux/2
  zero/1 -> Mux1/1, Mux1/2
  atmosphere/4 -> W/2

== system Citation/Cessna Citation 500/Citation model DASMAT/AIRCRAFT MODEL/LANDING GEAR ==
  note: Landing Gear Model
      | Cessna Citation 500
      | Version 0.04NLR
      | (c) A.R. Veldhuijzen September 2001
  x : Inport
  xdot : Inport  Port=2
  massinit : Inport  Port=3
  ua : Inport  Port=4
  terr elev : Inport  Port=5
  Gear axes-cg transformation : Subsystem
  Landing Gear model : Subsystem
  Switch : Switch  Threshold=0.95  SaturateOnIntegerOverflow=on
  gear position : Selector  IndexOptions=Index vector (dialog)  Indices=[8]  OutputSizes=1
  zero : Constant  Value=[0 0 0 0 0 0]
  Fmt : Outport
  wires:
  xdot/1 -> Landing Gear model/2(xdot)
  x/1 -> Landing Gear model/1(x), Gear axes-cg transformation/2("x ")
  massinit/1 -> Gear axes-cg transformation/3(massinit)
  Gear axes-cg transformation/1(FMt) -> Fmt/1
  zero/1 -> Switch/1
  Landing Gear model/1(Forces and Moments) -> Switch/3
  Switch/1 -> Gear axes-cg transformation/1(FMt model)
  ua/1 -> gear position/1
  gear position/1 -> Switch/2
  terr elev/1 -> Landing Gear model/3(terrain elevation)

== system Citation/Cessna Citation 500/Citation model DASMAT/AIRCRAFT MODEL/OBSERVATIONS ==
  note: Modified by Alex : Flight-Path Subsystem from Ac_mod instead of Ac_modpc
  x : Inport
  xdot : Inport  Port=2
  yuvw : Inport  Port=3
  FMtot : Inport  Port=4
  FMa : Inport  Port=5
  Fgr : Inport  Port=6
  massinit : Inport  Port=7
  yatm : Inport  Port=8
  Acceleration : Subsystem
  Energy : Subsystem
  Flight-Path : Subsystem
  yacc : Outport
  yfp : Outport  Port=2
  ys : Outport  Port=3
  wires:
  yuvw/1 -> Flight-Path/3(yuvw)
  Flight-Path/1(yfp) -> yfp/1
  Energy/1(ys) -> ys/1
  Acceleration/1(yacc) -> yacc/1
  FMa/1 -> Acceleration/4(FMa)
  Fgr/1 -> Acceleration/5(Fgr)
  yatm/1 -> Energy/3(yatm)
  FMtot/1 -> Acceleration/3(FMtot)
  Acceleration/2(acc earth) -> Flight-Path/4(acc earth)
  x/1 -> Flight-Path/1(x), Energy/1(x), Acceleration/1(x)
  xdot/1 -> Flight-Path/2(xdot), Energy/2(xdot), Acceleration/2(xdot)
  massinit/1 -> Acceleration/6(massinit)

== system Citation/Cessna Citation 500/Citation model DASMAT/AIRCRAFT MODEL/WIND/TURBULENCE ==
  "x " : Inport
  Logarithmic Wind model : Subsystem
  Mux : Mux  Inputs=[12 3]
  Vwind transformation : S-Function  FunctionName=ac_axes  Parameters=3  SFunctionDeploymentMode=off  EnableBusSupport=off
  wind : Outport
  wires:
  Mux/1 -> Vwind transformation/1
  Vwind transformation/1 -> wind/1
  "x "/1 -> Mux/1, Logarithmic Wind model/1(In1)
  Logarithmic Wind model/1(Out1) -> Mux/2

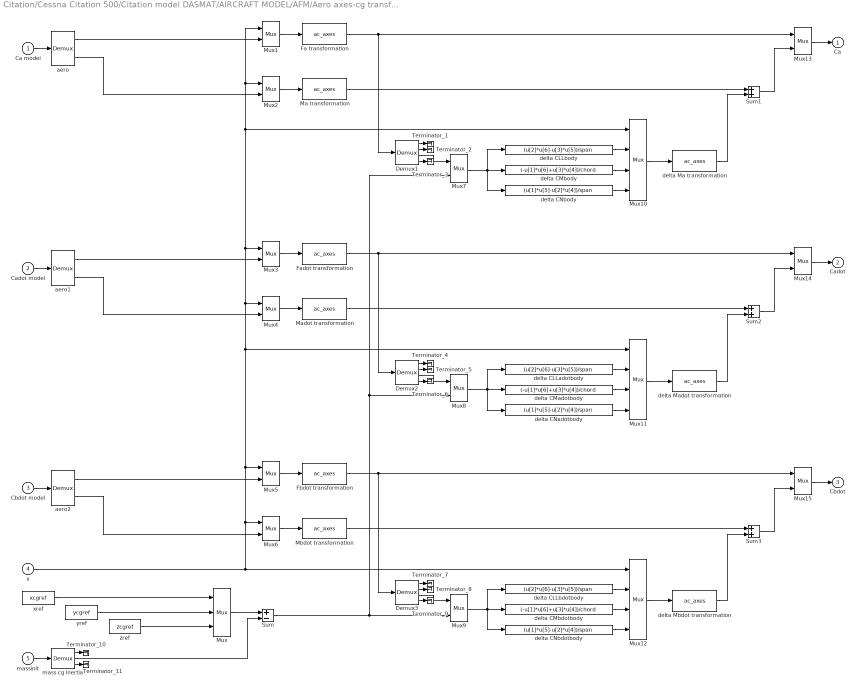
== system Citation/Cessna Citation 500/Citation model DASMAT/AIRCRAFT MODEL/AFM/Aero axes-cg transformation ==
  Ca model : Inport
  Cadot model : Inport  Port=2
  Cbdot model : Inport  Port=3
  "x " : Inport  Port=4
  massinit : Inport  Port=5
  Demux1 : Demux  Outputs=[3 3 3 3]
  Demux2 : Demux  Outputs=[3 3 3 3]
  Demux3 : Demux  Outputs=[3 3 3 3]
  Fa transformation : S-Function  FunctionName=ac_axes  Parameters=axes_CFMaero  SFunctionDeploymentMode=off  EnableBusSupport=off
  Fadot transformation : S-Function  FunctionName=ac_axes  Parameters=axes_CFMaero  SFunctionDeploymentMode=off  EnableBusSupport=off
  Fbdot transformation : S-Function  FunctionName=ac_axes  Parameters=axes_CFMaero  SFunctionDeploymentMode=off  EnableBusSupport=off
  Ma transformation : S-Function  FunctionName=ac_axes  Parameters=axes_CFMaero  SFunctionDeploymentMode=off  EnableBusSupport=off
  Madot transformation : S-Function  FunctionName=ac_axes  Parameters=axes_CFMaero  SFunctionDeploymentMode=off  EnableBusSupport=off
  Mbdot transformation : S-Function  FunctionName=ac_axes  Parameters=axes_CFMaero  SFunctionDeploymentMode=off  EnableBusSupport=off
  Mux : Mux  Inputs=3
  Mux{1..6} (6 alike) : Mux  Inputs=[12 3]
  Mux10 : Mux  Inputs=[12 1 1 1]
  Mux11 : Mux  Inputs=[12 1 1 1]
  Mux12 : Mux  Inputs=[12 1 1 1]
  Mux13 : Mux  Inputs=[12 12]
  Mux14 : Mux  Inputs=[12 12]
  Mux15 : Mux  Inputs=[12 12]
  Mux7 : Mux  Inputs=[3 3]
  Mux8 : Mux  Inputs=[3 3]
  Mux9 : Mux  Inputs=[3 3]
  Sum : Sum  Inputs=+-  SaturateOnIntegerOverflow=on  InputSameDT=on  OutDataTypeStr=Inherit: Same as first input
  Sum1 : Sum  SaturateOnIntegerOverflow=on  InputSameDT=on  OutDataTypeStr=Inherit: Same as first input
  Sum2 : Sum  SaturateOnIntegerOverflow=on  InputSameDT=on  OutDataTypeStr=Inherit: Same as first input
  Sum3 : Sum  SaturateOnIntegerOverflow=on  InputSameDT=on  OutDataTypeStr=Inherit: Same as first input
  Terminator_{1..11} (11 alike) : Terminator
  aero : Demux  Outputs=[3 3]
  aero1 : Demux  Outputs=[3 3]
  aero2 : Demux  Outputs=[3 3]
  delta CLLadotbody : Fcn  Expr=(u[2]*u[6]-u[3]*u[5])/span
  delta CLLbdotbody : Fcn  Expr=(u[2]*u[6]-u[3]*u[5])/span
  delta CLLbody : Fcn  Expr=(u[2]*u[6]-u[3]*u[5])/span
  delta CMadotbody : Fcn  Expr=(-u[1]*u[6]+u[3]*u[4])/chord
  delta CMbdotbody : Fcn  Expr=(-u[1]*u[6]+u[3]*u[4])/chord
  delta CMbody : Fcn  Expr=(-u[1]*u[6]+u[3]*u[4])/chord
  delta CNadotbody : Fcn  Expr=(u[1]*u[5]-u[2]*u[4])/span
  delta CNbdotbody : Fcn  Expr=(u[1]*u[5]-u[2]*u[4])/span
  delta CNbody : Fcn  Expr=(u[1]*u[5]-u[2]*u[4])/span
  delta Ma transformation : S-Function  FunctionName=ac_axes  Parameters=2  SFunctionDeploymentMode=off  EnableBusSupport=off
  delta Madot transformation : S-Function  FunctionName=ac_axes  Parameters=2  SFunctionDeploymentMode=off  EnableBusSupport=off
  delta Mbdot transformation : S-Function  FunctionName=ac_axes  Parameters=2  SFunctionDeploymentMode=off  EnableBusSupport=off
  mass cg inertia : Demux  Outputs=[1 3 4]
  xref : Constant  Value=xcgref
  yref : Constant  Value=ycgref
  zref : Constant  Value=zcgref
  Ca : Outport
  Cadot : Outport  Port=2
  Cbdot : Outport  Port=3
  wires:
  mass cg inertia/3 -> Terminator_11/1
  mass cg inertia/1 -> Terminator_10/1
  Demux3/4 -> Terminator_9/1
  Demux3/2 -> Terminator_8/1
  Demux3/1 -> Terminator_7/1
  Demux2/4 -> Terminator_6/1
  Demux2/2 -> Terminator_5/1
  Demux2/1 -> Terminator_4/1
  Demux1/4 -> Terminator_3/1
  Demux1/2 -> Terminator_2/1
  Demux1/1 -> Terminator_1/1
  aero1/1 -> Mux3/2
  Cadot model/1 -> aero1/1
  aero1/2 -> Mux4/2
  Ca model/1 -> aero/1
  massinit/1 -> mass cg inertia/1
  aero/1 -> Mux1/2
  xref/1 -> Mux/1
  yref/1 -> Mux/2
  zref/1 -> Mux/3
  mass cg inertia/2 -> Sum/2
  Mux/1 -> Sum/1
  Fa transformation/1 -> Demux1/1, Mux13/1
  Mux7/1 -> delta CLLbody/1, delta CNbody/1, delta CMbody/1
  delta CLLbody/1 -> Mux10/2
  delta CMbody/1 -> Mux10/3
  delta CNbody/1 -> Mux10/4
  Mux10/1 -> delta Ma transformation/1
  Ma transformation/1 -> Sum1/1
  Sum1/1 -> Mux13/2
  Mux13/1 -> Ca/1
  Mux1/1 -> Fa transformation/1
  Mux3/1 -> Fadot transformation/1
  Mux14/1 -> Cadot/1
  Sum2/1 -> Mux14/2
  Madot transformation/1 -> Sum2/1
  Mux12/1 -> delta Mbdot transformation/1
  delta CNbdotbody/1 -> Mux12/4
  delta CMbdotbody/1 -> Mux12/3
  delta CLLbdotbody/1 -> Mux12/2
  Mux9/1 -> delta CLLbdotbody/1, delta CNbdotbody/1, delta CMbdotbody/1
  Mux4/1 -> Madot transformation/1
  Mux2/1 -> Ma transformation/1
  aero/2 -> Mux2/2
  delta Ma transformation/1 -> Sum1/2
  Demux1/3 -> Mux7/1
  Demux3/3 -> Mux9/1
  Demux2/3 -> Mux8/1
  Mux11/1 -> delta Madot transformation/1
  delta CNadotbody/1 -> Mux11/4
  delta CMadotbody/1 -> Mux11/3
  delta CLLadotbody/1 -> Mux11/2
  Mux8/1 -> delta CLLadotbody/1, delta CNadotbody/1, delta CMadotbody/1
  Fadot transformation/1 -> Demux2/1, Mux14/1
  delta Madot transformation/1 -> Sum2/2
  Sum/1 -> Mux8/2, Mux7/2, Mux9/2
  Mux6/1 -> Mbdot transformation/1
  Mux5/1 -> Fbdot transformation/1
  aero2/2 -> Mux6/2
  Cbdot model/1 -> aero2/1
  aero2/1 -> Mux5/2
  "x "/1 -> Mux4/1, Mux3/1, Mux2/1, Mux1/1, Mux10/1, Mux11/1, Mux5/1, Mux6/1, Mux12/1
  Mbdot transformation/1 -> Sum3/1
  Fbdot transformation/1 -> Demux3/1, Mux15/1
  Sum3/1 -> Mux15/2
  delta Mbdot transformation/1 -> Sum3/2
  Mux15/1 -> Cbdot/1

== system Citation/Cessna Citation 500/Citation model DASMAT/AIRCRAFT MODEL/AFM/Aeromod ==
  x : Inport
  ua : Inport  Port=2
  massinit : Inport  Port=3
  yad1 : Inport  Port=4
  yad2 : Inport  Port=5
  gust : Inport  Port=6
  yatm : Inport  Port=7
  Demux : Demux  Outputs=[6 6 6 6]
  Mux1 : Mux  Inputs=24
  SubSystem : Subsystem
  cg selector : Selector  IndexOptions=Index vector (dialog)  Indices=[2 3 4]  OutputSizes=1
  Ca : Outport
  Cadot : Outport  Port=2
  Cbdot : Outport  Port=3
  Cag : Outport  Port=4
  wires:
  Mux1/1 -> Demux/1
  Demux/1 -> Ca/1
  Demux/2 -> Cadot/1
  Demux/3 -> Cbdot/1
  Demux/4 -> Cag/1
  SubSystem/2(CY) -> Mux1/2
  SubSystem/3(CZ) -> Mux1/3
  SubSystem/5(CM) -> Mux1/5
  SubSystem/6(CN) -> Mux1/6
  SubSystem/8(CYadot) -> Mux1/8
  SubSystem/9(CZadot) -> Mux1/9
  SubSystem/11(CMadot) -> Mux1/11
  SubSystem/12(CNadot) -> Mux1/12
  SubSystem/14(CYbdot) -> Mux1/14
  SubSystem/15(CZbdot) -> Mux1/15
  SubSystem/17(CMbdot) -> Mux1/17
  SubSystem/18(CNbdot) -> Mux1/18
  SubSystem/20(CYg) -> Mux1/20
  SubSystem/21(CZg) -> Mux1/21
  SubSystem/23(CMg) -> Mux1/23
  SubSystem/24(CNg) -> Mux1/24
  SubSystem/22(CLLg) -> Mux1/22
  SubSystem/19(CXg) -> Mux1/19
  SubSystem/16(CLLbdot) -> Mux1/16
  SubSystem/13(CXbdot) -> Mux1/13
  SubSystem/10(CLLadot) -> Mux1/10
  SubSystem/7(CXadot) -> Mux1/7
  SubSystem/4(CLL) -> Mux1/4
  SubSystem/1(CX) -> Mux1/1
  massinit/1 -> cg selector/1
  yad1/1 -> SubSystem/4(yad1)
  gust/1 -> SubSystem/6(gust)
  yad2/1 -> SubSystem/5(yad2)
  ua/1 -> SubSystem/2(ua)
  x/1 -> SubSystem/1(x)
  cg selector/1 -> SubSystem/3(cg)
  yatm/1 -> SubSystem/7(yatm)

== system Citation/Cessna Citation 500/Citation model DASMAT/AIRCRAFT MODEL/AFM/FMaerodims ==
  Ca : Inport
  Cadot : Inport  Port=2
  Cbdot : Inport  Port=3
  x : Inport  Port=4
  yad1 : Inport  Port=5
  Prod : Product  SaturateOnIntegerOverflow=on  InputSameDT=on  OutDataTypeStr=Inherit: Same as first input
  Prod1 : Product  Inputs=3  SaturateOnIntegerOverflow=on  InputSameDT=on  OutDataTypeStr=Inherit: Same as first input
  Prod2 : Product  Inputs=3  SaturateOnIntegerOverflow=on  InputSameDT=on  OutDataTypeStr=Inherit: Same as first input
  b/V : Fcn  Expr=span/u[4]
  c/V : Fcn  Expr=chord/u[4]
  dims : Subsystem
  dims1 : Subsystem
  dims2 : Subsystem
  qdyn*S : Fcn  Expr=u[2]*S
  FMa : Outport
  FMadot : Outport  Port=2
  FMbdot : Outport  Port=3
  wires:
  Ca/1 -> Prod/1
  Prod/1 -> dims/1(FM/length)
  dims/1(FM) -> FMa/1
  yad1/1 -> qdyn*S/1
  Cbdot/1 -> Prod2/1
  qdyn*S/1 -> Prod2/2, Prod1/2, Prod/2
  Cadot/1 -> Prod1/1
  Prod1/1 -> dims1/1(F FM/length)
  dims1/1(FM) -> FMadot/1
  Prod2/1 -> dims2/1(F FM/length)
  dims2/1(FM) -> FMbdot/1
  x/1 -> b/V/1, c/V/1
  c/V/1 -> Prod1/3
  b/V/1 -> Prod2/3

== system Citation/Cessna Citation 500/Citation model DASMAT/AIRCRAFT MODEL/AFM/FMgustdims ==
  Cag : Inport
  yad1 : Inport  Port=2
  Prod : Product  SaturateOnIntegerOverflow=on  InputSameDT=on  OutDataTypeStr=Inherit: Same as first input
  dims : Subsystem
  qdyn*S : Fcn  Expr=u[2]*S
  FMag : Outport
  wires:
  Cag/1 -> Prod/1
  Prod/1 -> dims/1(F M/length)
  yad1/1 -> qdyn*S/1
  dims/1(FM) -> FMag/1
  qdyn*S/1 -> Prod/2

== system Citation/Cessna Citation 500/Citation model DASMAT/AIRCRAFT MODEL/AFM/Gust axes-cg transformation ==
  Cag model : Inport
  "x " : Inport  Port=2
  massinit : Inport  Port=3
  Demux1 : Demux  Outputs=[3 3 3 3]
  Fag transformation : S-Function  FunctionName=ac_axes  Parameters=axes_CFMgust  SFunctionDeploymentMode=off  EnableBusSupport=off
  Mag transformation : S-Function  FunctionName=ac_axes  Parameters=axes_CFMgust  SFunctionDeploymentMode=off  EnableBusSupport=off
  Mux1 : Mux  Inputs=[12 3]
  Mux2 : Mux  Inputs=[12 3]
  Mux3 : Mux  Inputs=[3 3]
  Mux4 : Mux  Inputs=[12 1 1 1]
  Mux5 : Mux  Inputs=[12 12]
  Mux6 : Mux  Inputs=3
  Sum : Sum  Inputs=+-  SaturateOnIntegerOverflow=on  InputSameDT=on  OutDataTypeStr=Inherit: Same as first input
  Sum1 : Sum  SaturateOnIntegerOverflow=on  InputSameDT=on  OutDataTypeStr=Inherit: Same as first input
  Terminator_{1..5} (5 alike) : Terminator
  delta CLLbody : Fcn  Expr=(u[2]*u[6]-u[3]*u[5])/span
  delta CMbody : Fcn  Expr=(-u[1]*u[6]+u[3]*u[4])/chord
  delta CNbody : Fcn  Expr=(u[1]*u[5]-u[2]*u[4])/span
  delta Mag transformation : S-Function  FunctionName=ac_axes  Parameters=2  SFunctionDeploymentMode=off  EnableBusSupport=off
  gust : Demux  Outputs=[3 3]
  mass cg inertia : Demux  Outputs=[1 3 4]
  xref : Constant  Value=xcgref
  yref : Constant  Value=ycgref
  zref : Constant  Value=zcgref
  Cag : Outport
  wires:
  mass cg inertia/3 -> Terminator_5/1
  mass cg inertia/1 -> Terminator_4/1
  Demux1/4 -> Terminator_3/1
  Demux1/2 -> Terminator_2/1
  Demux1/1 -> Terminator_1/1
  Cag model/1 -> gust/1
  massinit/1 -> mass cg inertia/1
  gust/1 -> Mux1/2
  xref/1 -> Mux6/1
  yref/1 -> Mux6/2
  zref/1 -> Mux6/3
  mass cg inertia/2 -> Sum/2
  Mux6/1 -> Sum/1
  Fag transformation/1 -> Demux1/1, Mux5/1
  Mag transformation/1 -> Sum1/1
  Sum1/1 -> Mux5/2
  Mux5/1 -> Cag/1
  Mux1/1 -> Fag transformation/1
  delta Mag transformation/1 -> Sum1/2
  Mux2/1 -> Mag transformation/1
  Sum/1 -> Mux3/2
  gust/2 -> Mux2/2
  "x "/1 -> Mux2/1, Mux1/1, Mux4/1
  Mux3/1 -> delta CLLbody/1, delta CNbody/1, delta CMbody/1
  delta CLLbody/1 -> Mux4/2
  delta CMbody/1 -> Mux4/3
  delta CNbody/1 -> Mux4/4
  Demux1/3 -> Mux3/1
  Mux4/1 -> delta Mag transformation/1

== system Citation/Cessna Citation 500/Citation model DASMAT/AIRCRAFT MODEL/EFM/Engine axes-cg transformation ==
  FMt model : Inport
  "x " : Inport  Port=2
  massinit : Inport  Port=3
  Demux : Demux  Outputs=[3 3 3 3]
  Ft transformation : S-Function  FunctionName=ac_axes  Parameters=2  SFunctionDeploymentMode=off  EnableBusSupport=off
  Mt transformation : S-Function  FunctionName=ac_axes  Parameters=2  SFunctionDeploymentMode=off  EnableBusSupport=off
  Mux1 : Mux  Inputs=[12 3]
  Mux2 : Mux  Inputs=[12 3]
  Mux3 : Mux  Inputs=[3 3]
  Mux4 : Mux  Inputs=[12 1 1 1]
  Mux5 : Mux  Inputs=[12 12]
  "Neg " : Gain  Gain=-1  SaturateOnIntegerOverflow=on  OutDataTypeStr=Inherit: Same as input  ParamDataTypeStr=Inherit: Same as input
  Sum1 : Sum  SaturateOnIntegerOverflow=on  InputSameDT=on  OutDataTypeStr=Inherit: Same as first input
  Terminator_{1..5} (5 alike) : Terminator
  delta LLbody : Fcn  Expr=u[2]*u[6]-u[3]*u[5]
  delta Mbody : Fcn  Expr=-u[1]*u[6]+u[3]*u[4]
  delta Mt transformation : S-Function  FunctionName=ac_axes  Parameters=2  SFunctionDeploymentMode=off  EnableBusSupport=off
  delta Nbody : Fcn  Expr=u[1]*u[5]-u[2]*u[4]
  engine : Demux  Outputs=[3 3]
  mass cg inertia : Demux  Outputs=[1 3 4]
  FMt : Outport
  wires:
  mass cg inertia/3 -> Terminator_5/1
  mass cg inertia/1 -> Terminator_4/1
  Demux/4 -> Terminator_3/1
  Demux/2 -> Terminator_2/1
  Demux/1 -> Terminator_1/1
  FMt model/1 -> engine/1
  massinit/1 -> mass cg inertia/1
  engine/1 -> Mux1/2
  Ft transformation/1 -> Demux/1, Mux5/1
  Mt transformation/1 -> Sum1/1
  Sum1/1 -> Mux5/2
  Mux5/1 -> FMt/1
  Mux1/1 -> Ft transformation/1
  delta Mt transformation/1 -> Sum1/2
  Mux2/1 -> Mt transformation/1
  engine/2 -> Mux2/2
  "x "/1 -> Mux2/1, Mux1/1, Mux4/1
  Mux3/1 -> delta LLbody/1, delta Nbody/1, delta Mbody/1
  delta LLbody/1 -> Mux4/2
  delta Mbody/1 -> Mux4/3
  delta Nbody/1 -> Mux4/4
  Mux4/1 -> delta Mt transformation/1
  Demux/3 -> Mux3/1
  mass cg inertia/2 -> "Neg "/1
  "Neg "/1 -> Mux3/2

== system Citation/Cessna Citation 500/Citation model DASMAT/AIRCRAFT MODEL/EFM/Engmod ==
  x : Inport
  ut : Inport  Port=2
  yatm : Inport  Port=3
  yad1 : Inport  Port=4
  yad2 : Inport  Port=5
  Citation eng_mod : Subsystem
  Mux : Mux  Inputs=[12 2 8 2 8]
  FMt : Outport
  ypp : Outport  Port=2
  wires:
  x/1 -> Mux/1
  ut/1 -> Mux/2
  yatm/1 -> Mux/3
  yad1/1 -> Mux/4
  yad2/1 -> Mux/5
  Mux/1 -> Citation eng_mod/1(In1)
  Citation eng_mod/1(Out1) -> FMt/1
  Citation eng_mod/2(ypp) -> ypp/1
